simulink model "Bai28"  (R2020a)
settings: Solver=VariableStepAuto  StartTime=0.0  StopTime=10.0  RelTol=1e-3
settings Model: Creator=NgocNguyen  LastModifiedBy=NgocNguyen

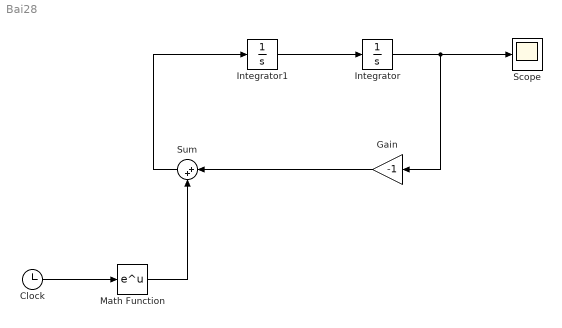
== system Bai28 ==
  Clock : Clock
  Gain : Gain  Gain=-1
  Integrator : Integrator
  Integrator1 : Integrator  InitialCondition=1
  Math Function : Math  SaturateOnIntegerOverflow=on
  Scope : Scope
  Sum : Sum  Inputs=|++
  wires:
  Integrator/1 -> Gain/1, Scope/1
  Integrator1/1 -> Integrator/1
  Gain/1 -> Sum/1
  Math Function/1 -> Sum/2
  Sum/1 -> Integrator1/1
  Clock/1 -> Math Function/1
